simulink model "robot_capteur_etu"  (R2022b)
settings: Solver=VariableStepAuto  StartTime=0.0  StopTime=10.0  RelTol=1e-3
values from neighbouring files (symbols this model uses):
  K = [0.67 19.9055 1.0747  1.9614]    [simu_robot_etu.m]
  ue = 0    [simu_robot_etu.m]
  x0 = [0 pi/10 0 0]'    [simu_robot_etu.m]
  xe = [0 0 0 0]'    [simu_robot_etu.m]
settings Model: Creator=felix  LastModifiedBy=felix

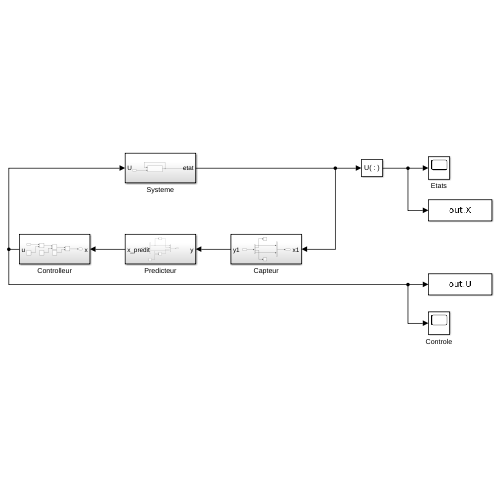
[thumbnail: Simulink's stored preview of the top-level diagram]
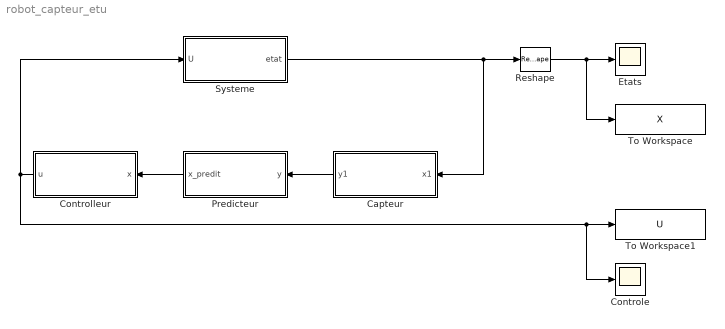
== system robot_capteur_etu ==
  Capteur : Subsystem
  Controle : Scope
  Controlleur : Subsystem
  Etats : Scope
  Predicteur : Subsystem
  Reshape : Reshape
  Systeme : Subsystem
  To Workspace : ToWorkspace  VariableName=X  SaveFormat=Timeseries  SampleTime=-1
  To Workspace1 : ToWorkspace  VariableName=U  SaveFormat=Timeseries  SampleTime=-1
  wires:
  Controlleur/1(u) -> Systeme/1(U), Controle/1, To Workspace1/1
  Reshape/1 -> To Workspace/1, Etats/1
  Systeme/1(etat) -> Capteur/1(x1), Reshape/1
  Predicteur/1(x_predit) -> Controlleur/1(x)
  Capteur/1(y1) -> Predicteur/1(y)

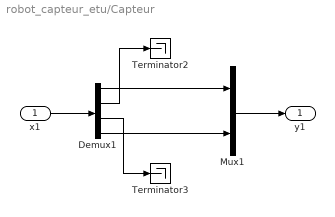
== system robot_capteur_etu/Capteur ==
  x1 : Inport
  Demux1 : Demux
  Mux1 : Mux  Inputs=2
  Terminator2 : Terminator
  Terminator3 : Terminator
  y1 : Outport
  wires:
  Demux1/4 -> Mux1/2
  Mux1/1 -> y1/1
  x1/1 -> Demux1/1
  Demux1/2 -> Terminator2/1
  Demux1/1 -> Mux1/1
  Demux1/3 -> Terminator3/1

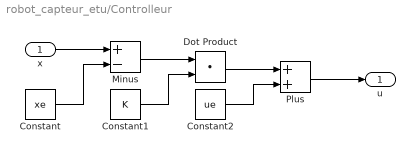
== system robot_capteur_etu/Controlleur ==
  x : Inport
  Constant : Constant  Value=xe
  Constant1 : Constant  Value=K  VectorParams1D=off
  Constant2 : Constant  Value=ue
  Dot Product : DotProduct  OutDataTypeStr=Inherit: Inherit via internal rule
  Minus : Sum  Inputs=+-
  Plus : Sum
  u : Outport
  wires:
  x/1 -> Minus/1
  Constant/1 -> Minus/2
  Minus/1 -> Dot Product/1
  Constant1/1 -> Dot Product/2
  Dot Product/1 -> Plus/1
  Constant2/1 -> Plus/2
  Plus/1 -> u/1

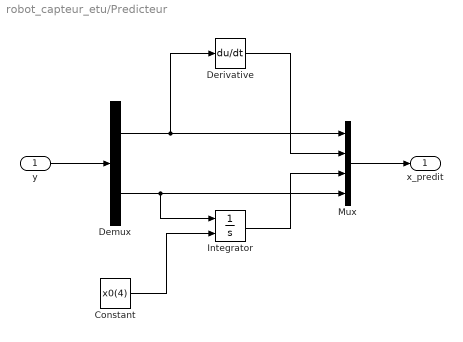
== system robot_capteur_etu/Predicteur ==
  y : Inport
  Constant : Constant  Value=x0(4)
  Demux : Demux  Outputs=2
  Derivative : Derivative
  Integrator : Integrator  InitialConditionSource=external
  Mux : Mux
  x_predit : Outport
  wires:
  y/1 -> Demux/1
  Demux/2 -> Integrator/1, Mux/4
  Constant/1 -> Integrator/2
  Mux/1 -> x_predit/1
  Integrator/1 -> Mux/3
  Demux/1 -> Mux/1, Derivative/1
  Derivative/1 -> Mux/2

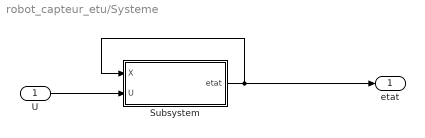
== system robot_capteur_etu/Systeme ==
  U : Inport
  Subsystem : Subsystem
  etat : Outport
  wires:
  U/1 -> Subsystem/2(U)
  Subsystem/1(etat) -> Subsystem/1(X), etat/1

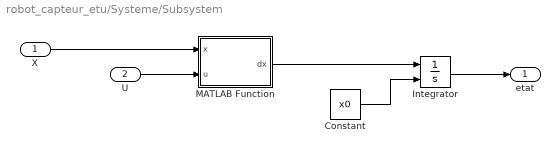
== system robot_capteur_etu/Systeme/Subsystem ==
  X : Inport
  U : Inport  Port=2
  Constant : Constant  Value=x0
  Integrator : Integrator  InitialConditionSource=external
  MATLAB Function : MATLAB Function  TreatAsAtomicUnit=on
  etat : Outport
  wires:
  Integrator/1 -> etat/1
  MATLAB Function/1(dx) -> Integrator/1
  Constant/1 -> Integrator/2
  U/1 -> MATLAB Function/2(u)
  X/1 -> MATLAB Function/1(x)

== matlab function robot_capteur_etu/Systeme/Subsystem/MATLAB Function ==
  data: x input; u input; dx output
function dx   = fonction( x, u)
%   Dynamic equations of motion of the segway on an axis.
%   Inputs: - x = [theta psi dtheta dpsi]
%               theta: average angle of the wheels      [rad]
%               psi: body pitch angle                   [rad]
%               dtheta: average velocity of the wheels  [rad/s]
%               dpsi: body pitch velocity               [rad/s]
%          - u: DC motor voltage (same value for both motors) [V]

    % State
    psi = x(2);
    dtheta = x(3);
    dpsi = x(4);

    % Parameters
    
    g = 9.81;           % gravity acceleration [m/sec^2]
    m = 0.03;           % wheel weight [kg]
    R = 0.04;           % wheel radius [m]
    Jw = m*R^2/2;       % wheel inertia moment [kg*m^2]
    M = 0.6;            % body weight [kg]
    H = 0.144;          % body height [m]
    L = H/2;            % distance of the center of mass from the wheel axle [m]
    Jpsi = M*L^2/3;     % body pitch inertia [kgm^2]
    Jm = 1e-5;          % DC motor inertia moment [kgm^2]
    Rm = 6.69;          % DC motor resistance [Ohm]
    Kb = 0.468;         % DC motor back EMF constant [Vsec/rad]
    Kt = 0.317;         % DC motor torque constant [Nm/A]
    n = 1;              % gear ratio
    fm = 0.0022;        % friction coefficient between body and DC motor
    fw = 0;             % friction coefficient between wheel and floor
    
    % Equations of motion
    c1 = (2*m+M)*R^2 + 2*Jw + 2*n^2*Jm;
    c2 = M*L*R*cos(psi) - 2*n^2*Jm;
    c3 = -M*L*R*dpsi^2*sin(psi);
    c4 = M*L^2 + Jpsi + 2*n^2*Jm;
    c5 = -M*g*L*sin(psi);

    alpha = Kt/Rm;
    beta = Kt*Kb/Rm + fm;

    Ftheta = alpha*(2*u) - 2*(beta+fw)*dtheta + 2*beta*dpsi;
    Fpsi = -alpha*(2*u) + 2*beta*dtheta - 2*beta*dpsi;

    ddtheta = (c4*c3 - c2*c5 + c4*Ftheta - c2*Fpsi)/(c4*c1 - c2^2);
    ddpsi = (Fpsi- c2*ddtheta - c5)/c4;
    dx = [dtheta dpsi ddtheta ddpsi]';

end
